simulink model "Mdl_Gear"  (R2024b)
settings: Solver=FixedStepDiscrete  StartTime=0.0  StopTime=10.0  FixedStep=0.1  RelTol=1e-3  EnableMultiTasking=on
values from neighbouring files (symbols this model uses):
  GEAR_MODE_OFF = mpt.Parameter    [Mdl_Gear_DD.m]
  GEAR_STATUS_OFF = mpt.Parameter    [Mdl_Gear_DD.m]
  HMI_READY = mpt.Parameter    [Mdl_Gear_DD.m]
  IND_FLASH_1HZ = mpt.Parameter    [Mdl_Gear_DD.m]
  IND_FLASH_4HZ = mpt.Parameter    [Mdl_Gear_DD.m]
  IND_TURN_OFF = mpt.Parameter    [Mdl_Gear_DD.m]
  Init_Count = mpt.Parameter    [Mdl_Gear_DD.m]
  Mdl_Gear_cTaskPeriod = mpt.Parameter    [Mdl_Gear_rte_types.m]
  PGM_LOGIC_ENABLE = mpt.Parameter    [Mdl_Gear_DD.m]
  RTE_E_MAX_AGE_EXCEEDED = mpt.Parameter    [Mdl_Gear_rte_types.m]
  RTE_E_NEVER_RECEIVED = mpt.Parameter    [Mdl_Gear_rte_types.m]
  Shift_Blink_P1 = mpt.Parameter    [Mdl_Gear_DD.m]
  Shift_Blink_P2 = mpt.Parameter    [Mdl_Gear_DD.m]
  STATUS_OFF = mpt.Parameter    [Mdl_Gear_DD.m]
  STATUS_ON = mpt.Parameter    [Mdl_Gear_DD.m]
  Timer_Param = mpt.Parameter    [Mdl_Gear_DD.m]
  TYPE1 = mpt.Parameter    [Mdl_Gear_DD.m]
  TYPE1_SBW = mpt.Parameter    [Mdl_Gear_DD.m]
  TYPE2 = mpt.Parameter    [Mdl_Gear_DD.m]
  TYPE2_MECH = mpt.Parameter    [Mdl_Gear_DD.m]
  TYPE3 = mpt.Parameter    [Mdl_Gear_DD.m]
  VALUE_FIFTEEN = mpt.Parameter    [Mdl_Gear_DD.m]
  VALUE_FIVE = mpt.Parameter    [Mdl_Gear_DD.m]
  VALUE_FOUR = mpt.Parameter    [Mdl_Gear_DD.m]
  VALUE_ONE = mpt.Parameter    [Mdl_Gear_DD.m]
  VALUE_TEN = mpt.Parameter    [Mdl_Gear_DD.m]
  VALUE_THREE = mpt.Parameter    [Mdl_Gear_DD.m]
  VALUE_TWO = mpt.Parameter    [Mdl_Gear_DD.m]
  VALUE_ZERO = mpt.Parameter    [Mdl_Gear_DD.m]
undefined symbols (not defined in the file or in its folder): CLUSTER_INACTIVE, eGearIn, eGearModeIn, eGearRecommendationIn, eGearStatusIn, eSIGNAL_MISSING, eSIGNAL_NEVER_RECEIVED, IgnOff, IgnOn, NETWORK_NORMAL, NETWORK_STANDALONE, PTSYS_EV, PTSYS_PHV, tRxSignalId_type_instance, tRxSignalStatus_type_instance
libraries: simulink x9
(part 2 of 2)

== matlab function Mdl_Gear/Mdl_Gear_Task_sys/Subsystem/Subsystem1/Subsystem/Display Blink Effect Determination ==
  data: Vehicle_status input; GearStatus_Val input; IND_FLASH_4HZ parameter; IND_FLASH_1HZ parameter; Shift_Blink_Pattern output; IND_TURN_OFF parameter; Shift_Blink_P2 parameter; Shift_Blink_P1 parameter; GEAR_MODE_OFF parameter; GearStatus_Sts input; eSIGNAL_NEVER_RECEIVED parameter; eSIGNAL_MISSING parameter; Prev_Shift_Blink_Pattern input; NETWORK_STANDALONE parameter
function Shift_Blink_Pattern = fcn(Vehicle_status, GearStatus_Val, IND_FLASH_4HZ, IND_FLASH_1HZ, IND_TURN_OFF, Shift_Blink_P2, Shift_Blink_P1, GEAR_MODE_OFF, GearStatus_Sts, eSIGNAL_NEVER_RECEIVED, eSIGNAL_MISSING, Prev_Shift_Blink_Pattern, NETWORK_STANDALONE)

aVarTruthTableCondition_1 = false;
aVarTruthTableCondition_2 = false;
aVarTruthTableCondition_3 = false;
aVarTruthTableCondition_4 = false;


% Appmode is Standalone or  CAN status is never recived

aVarTruthTableCondition_1 = logical(((Vehicle_status == NETWORK_STANDALONE ) || ( GearStatus_Sts == eSIGNAL_NEVER_RECEIVED)));

% Blink_Pattern Off

aVarTruthTableCondition_2 = logical(( GearStatus_Sts== eSIGNAL_MISSING));

% Blink Pattern 1

aVarTruthTableCondition_3 = logical(GearStatus_Val== Shift_Blink_P1);

% Blink Pattern 2

aVarTruthTableCondition_4 = logical(GearStatus_Val== Shift_Blink_P2);

if (aVarTruthTableCondition_1)
    aFcnTruthTableAction_4();
elseif (aVarTruthTableCondition_2)
    aFcnTruthTableAction_1();
elseif (aVarTruthTableCondition_3)
    aFcnTruthTableAction_2();
elseif (aVarTruthTableCondition_4)
    aFcnTruthTableAction_3();
else % Default
    aFcnTruthTableAction_1();
end

function aFcnTruthTableAction_1()

% Shift Blink OFF

Shift_Blink_Pattern = IND_TURN_OFF;

function aFcnTruthTableAction_2()

% Shift Blink Pattern 1 as 1 Hz

Shift_Blink_Pattern = IND_FLASH_1HZ;

function aFcnTruthTableAction_3()

% Shift Blink Pattern 2 as 4 hz

Shift_Blink_Pattern = IND_FLASH_4HZ;

function aFcnTruthTableAction_4()

% No change

Shift_Blink_Pattern = Prev_Shift_Blink_Pattern;

== matlab function Mdl_Gear/Mdl_Gear_Task_sys/Subsystem/Subsystem1/Subsystem/Determination of Shift Up ==
  data: Vehicle_status input; Shift_Up_Ind output; STATUS_OFF parameter; Shift_Up_Can_Value input; Shift_Up_Can_Status input; NETWORK_NORMAL parameter; NETWORK_STANDALONE parameter; eSIGNAL_NEVER_RECEIVED parameter; eSIGNAL_MISSING parameter; Prev_Shift_Up_Ind input; VALUE_ONE parameter; VALUE_FIFTEEN parameter; STATUS_ON parameter
function Shift_Up_Ind = fcn(Vehicle_status, STATUS_OFF, Shift_Up_Can_Value, Shift_Up_Can_Status, NETWORK_NORMAL, NETWORK_STANDALONE, eSIGNAL_NEVER_RECEIVED, eSIGNAL_MISSING, Prev_Shift_Up_Ind, VALUE_ONE, VALUE_FIFTEEN, STATUS_ON)

aVarTruthTableCondition_1 = false;
aVarTruthTableCondition_2 = false;
aVarTruthTableCondition_3 = false;


% Appmode is Standalone or  CAN status is never recived

aVarTruthTableCondition_1 = logical(((Vehicle_status == NETWORK_STANDALONE ) || ( Shift_Up_Can_Status == eSIGNAL_NEVER_RECEIVED)));

% CAN status is Missing

aVarTruthTableCondition_2 = logical((Shift_Up_Can_Status == eSIGNAL_MISSING));

% Shift Up CAN value is 1

aVarTruthTableCondition_3 = logical((Shift_Up_Can_Value == VALUE_ONE));

if (aVarTruthTableCondition_1)
    aFcnTruthTableAction_2();
elseif (aVarTruthTableCondition_2)
    aFcnTruthTableAction_1();
elseif (aVarTruthTableCondition_3)
    aFcnTruthTableAction_3();
else % Default
    aFcnTruthTableAction_1();
end

function aFcnTruthTableAction_1()

% Shift up is Off

Shift_Up_Ind = STATUS_OFF;

function aFcnTruthTableAction_2()

% Previous Step Up

Shift_Up_Ind = Prev_Shift_Up_Ind;

function aFcnTruthTableAction_3()

% Shift up is On

Shift_Up_Ind = STATUS_ON;

== matlab function Mdl_Gear/Mdl_Gear_Task_sys/Subsystem/Subsystem1/Subsystem/Determination of Shift Down ==
  data: Vehicle_status input; Shift_Down_Ind output; STATUS_OFF parameter; Shift_Down_Can_Value input; Shift_Down_Can_Status input; NETWORK_NORMAL parameter; NETWORK_STANDALONE parameter; eSIGNAL_NEVER_RECEIVED parameter; eSIGNAL_MISSING parameter; Prev_Shift_Down_Ind input; VALUE_TWO parameter; VALUE_FIFTEEN parameter; STATUS_ON parameter
function Shift_Down_Ind = fcn(Vehicle_status, STATUS_OFF, Shift_Down_Can_Value, Shift_Down_Can_Status, NETWORK_NORMAL, NETWORK_STANDALONE, eSIGNAL_NEVER_RECEIVED, eSIGNAL_MISSING, Prev_Shift_Down_Ind, VALUE_TWO, VALUE_FIFTEEN, STATUS_ON)

aVarTruthTableCondition_1 = false;
aVarTruthTableCondition_2 = false;
aVarTruthTableCondition_3 = false;


% Appmode is Standalone or  CAN status is never recived

aVarTruthTableCondition_1 = logical(((Vehicle_status == NETWORK_STANDALONE ) || ( Shift_Down_Can_Status == eSIGNAL_NEVER_RECEIVED)));

% CAN status is Missing

aVarTruthTableCondition_2 = logical((Shift_Down_Can_Status == eSIGNAL_MISSING));

% Shift down CAN value is 1

aVarTruthTableCondition_3 = logical((Shift_Down_Can_Value == VALUE_TWO));

if (aVarTruthTableCondition_1)
    aFcnTruthTableAction_2();
elseif (aVarTruthTableCondition_2)
    aFcnTruthTableAction_1();
elseif (aVarTruthTableCondition_3)
    aFcnTruthTableAction_3();
else % Default
    aFcnTruthTableAction_1();
end

function aFcnTruthTableAction_1()

% Shift down status is Off

Shift_Down_Ind = STATUS_OFF;

function aFcnTruthTableAction_2()

% Previous Shift down status

Shift_Down_Ind = Prev_Shift_Down_Ind;

function aFcnTruthTableAction_3()

% Shift down status is On

Shift_Down_Ind = STATUS_ON;

== matlab function Mdl_Gear/Mdl_Gear_Task_sys/Subsystem/Subsystem1/Subsystem/Determination of Display deceleration state ==
  data: Vehicle_status input; PTSys_flag input; DisplayDecState output; STATUS_OFF parameter; SFT_MET_Value input; SFT_MET_Status input; CLDCLV_Value input; CLDCLV_Status input; NETWORK_NORMAL parameter; NETWORK_STANDALONE parameter; RTE_E_NEVER_RECEIVED parameter; RTE_E_MAX_AGE_EXCEEDED parameter; Prev_DisplayDecState input; VALUE_ONE parameter; VALUE_TWO parameter; VALUE_ZERO parameter; VALUE_THREE parameter; VALUE_FOUR parameter; VALUE_FIVE parameter; PTSYS_PHV parameter; PTSYS_EV parameter
function DisplayDecState = fcn(Vehicle_status, PTSys_flag, STATUS_OFF, SFT_MET_Value, SFT_MET_Status, CLDCLV_Value, CLDCLV_Status, NETWORK_NORMAL, NETWORK_STANDALONE, RTE_E_NEVER_RECEIVED, RTE_E_MAX_AGE_EXCEEDED, Prev_DisplayDecState, VALUE_ONE, VALUE_TWO, VALUE_ZERO, VALUE_THREE, VALUE_FOUR, VALUE_FIVE, PTSYS_PHV, PTSYS_EV)

aVarTruthTableCondition_1 = false;
aVarTruthTableCondition_2 = false;
aVarTruthTableCondition_3 = false;
aVarTruthTableCondition_4 = false;
aVarTruthTableCondition_5 = false;
aVarTruthTableCondition_6 = false;
aVarTruthTableCondition_7 = false;
aVarTruthTableCondition_8 = false;


% Check App mode is Standalone

aVarTruthTableCondition_1 = logical((Vehicle_status == NETWORK_STANDALONE ));

% Check PTsys flag and SFT_MET value is other than 4 and 5

aVarTruthTableCondition_2 = logical((((PTSys_flag ~= PTSYS_PHV) && (PTSys_flag ~= PTSYS_EV)) || ((SFT_MET_Value ~= VALUE_FOUR) && ( SFT_MET_Value ~= VALUE_FIVE))));

% Missing and Never received

aVarTruthTableCondition_3 = logical((CLDCLV_Status == RTE_E_NEVER_RECEIVED) || (CLDCLV_Status == RTE_E_MAX_AGE_EXCEEDED) || (SFT_MET_Status == RTE_E_NEVER_RECEIVED) || (SFT_MET_Status == RTE_E_MAX_AGE_EXCEEDED));

% CANSignal  CLDCLV is 1

aVarTruthTableCondition_4 = logical((CLDCLV_Value == VALUE_ONE));

% CANSignal  CLDCLV is 2

aVarTruthTableCondition_5 = logical((CLDCLV_Value == VALUE_TWO));

% CANSignal  CLDCLV is 3

aVarTruthTableCondition_6 = logical((CLDCLV_Value == VALUE_THREE));

% CANSignal  CLDCLV is 4

aVarTruthTableCondition_7 = logical((CLDCLV_Value == VALUE_FOUR));

% CANSignal  CLDCLV is 5

aVarTruthTableCondition_8 = logical((CLDCLV_Value == VALUE_FIVE));

if (aVarTruthTableCondition_1)
    aFcnTruthTableAction_2();
elseif (aVarTruthTableCondition_2)
    aFcnTruthTableAction_1();
elseif (aVarTruthTableCondition_3)
    aFcnTruthTableAction_1();
elseif (aVarTruthTableCondition_4)
    aFcnTruthTableAction_3();
elseif (aVarTruthTableCondition_5)
    aFcnTruthTableAction_4();
elseif (aVarTruthTableCondition_6)
    aFcnTruthTableAction_5();
elseif (aVarTruthTableCondition_7)
    aFcnTruthTableAction_6();
elseif (aVarTruthTableCondition_8)
    aFcnTruthTableAction_7();
else % Default
    aFcnTruthTableAction_1();
end

function aFcnTruthTableAction_1()

% Off state

DisplayDecState = STATUS_OFF;

function aFcnTruthTableAction_2()

% Previous state

DisplayDecState = Prev_DisplayDecState;

function aFcnTruthTableAction_3()

% LEVEL_0

DisplayDecState = VALUE_ONE;

function aFcnTruthTableAction_4()

% LEVEL_1

DisplayDecState = VALUE_TWO;

function aFcnTruthTableAction_5()

% LEVEL_2

DisplayDecState = VALUE_THREE;

function aFcnTruthTableAction_6()

% LEVEL_3

DisplayDecState = VALUE_FOUR;

function aFcnTruthTableAction_7()

% LEVEL_4

DisplayDecState = VALUE_FIVE;

== matlab function Mdl_Gear/Mdl_Gear_Task_sys/Subsystem/Subsystem1/Subsystem/Output of GUI_SHIFT_TYPE ==
  data: DisplayDecState input; Screen_ShiftType output; STATUS_OFF parameter; Shift_Up_Ind input; Shift_Down_Ind input; VALUE_ONE parameter; VALUE_FIFTEEN parameter; VALUE_FIVE parameter; TYPE1 parameter; TYPE2 parameter; TYPE3 parameter; STATUS_ON parameter
function Screen_ShiftType = fcn(DisplayDecState, STATUS_OFF, Shift_Up_Ind, Shift_Down_Ind, VALUE_ONE, VALUE_FIFTEEN, VALUE_FIVE, TYPE1, TYPE2, TYPE3, STATUS_ON)

aVarTruthTableCondition_1 = false;
aVarTruthTableCondition_2 = false;


% Display Deceleration status is Off and Shift up or Down is On

aVarTruthTableCondition_1 = logical(((DisplayDecState == STATUS_OFF)  && ((Shift_Up_Ind == STATUS_ON) || (Shift_Down_Ind == STATUS_ON))));

% Display Deceleration status is 1 to 5

aVarTruthTableCondition_2 = logical(((DisplayDecState >= VALUE_ONE) && (DisplayDecState <= VALUE_FIVE)));

if (aVarTruthTableCondition_1)
    aFcnTruthTableAction_2();
elseif (aVarTruthTableCondition_2)
    aFcnTruthTableAction_3();
else % Default
    aFcnTruthTableAction_1();
end

function aFcnTruthTableAction_1()

% Screen Shift type is TYPE1

Screen_ShiftType = TYPE1;

function aFcnTruthTableAction_2()

% Screen Shift type is TYPE2

Screen_ShiftType = TYPE2;

function aFcnTruthTableAction_3()

% Screen Shift type is TYPE3

Screen_ShiftType = TYPE3;

== matlab function Mdl_Gear/Mdl_Gear_Task_sys/Subsystem/Subsystem1/Subsystem/Determination of Shift Position and Shift Mode and Gear Step ==
  data: GEAR_STATUS_OFF parameter; Shift_Position input; Shift_Ind_Pos output uint8; Gear_Step input; Shift_Pos_RANGE_P parameter; Shift_Pos_RANGE_R parameter; Shift_Pos_RANGE_N parameter; Shift_Pos_RANGE_B parameter; Shift_Pos_RANGE_SD parameter; Shift_Pos_RANGE_D parameter; Shift_Pos_RANGE_S parameter; Shift_Pos_RANGE_M parameter; Shift_PosInd_Ind_S parameter; Shift_PosInd_Ind_M parameter; Shift_PosInd_Ind_D parameter; Shift_PosInd_P parameter; Shift_PosInd_R parameter; Shift_PosInd_N parameter; Shift_PosInd_D parameter; Shift_PosInd_B parameter; Shift_PosInd_SD parameter; Shift_PosInd_M parameter; Shift_PosInd_S parameter; GEAR_STATUS_ON parameter; Gear_Flag output uint8
function [Shift_Ind_Pos, Gear_Flag] = fcn(GEAR_STATUS_OFF, Shift_Position, Gear_Step, Shift_Pos_RANGE_P, Shift_Pos_RANGE_R, Shift_Pos_RANGE_N, Shift_Pos_RANGE_B, Shift_Pos_RANGE_SD, Shift_Pos_RANGE_D, Shift_Pos_RANGE_S, Shift_Pos_RANGE_M, Shift_PosInd_Ind_S, Shift_PosInd_Ind_M, Shift_PosInd_Ind_D, Shift_PosInd_P, Shift_PosInd_R, Shift_PosInd_N, Shift_PosInd_D, Shift_PosInd_B, Shift_PosInd_SD, Shift_PosInd_M, Shift_PosInd_S, GEAR_STATUS_ON)

aVarTruthTableCondition_1 = false;
aVarTruthTableCondition_2 = false;
aVarTruthTableCondition_3 = false;
aVarTruthTableCondition_4 = false;
aVarTruthTableCondition_5 = false;
aVarTruthTableCondition_6 = false;
aVarTruthTableCondition_7 = false;
aVarTruthTableCondition_8 = false;
aVarTruthTableCondition_9 = false;
aVarTruthTableCondition_10 = false;
aVarTruthTableCondition_11 = false;
aVarTruthTableCondition_12 = false;
aVarTruthTableCondition_13 = false;


% Shift Position Determination Range P,R,N,B,SD and Gear Step >0

aVarTruthTableCondition_1 = logical(((Shift_Position == Shift_Pos_RANGE_P)||(Shift_Position == Shift_Pos_RANGE_N)||(Shift_Position == Shift_Pos_RANGE_R)|| (Shift_Position == Shift_Pos_RANGE_B)||(Shift_Position == Shift_Pos_RANGE_SD)) &&(Gear_Step == GEAR_STATUS_OFF));

% Shift Position Determination Range P and Gear Step ==0

aVarTruthTableCondition_2 = logical((Shift_Position== Shift_Pos_RANGE_P));

% Shift Position Determination Range R and Gear Step ==0

aVarTruthTableCondition_3 = logical((Shift_Position == Shift_Pos_RANGE_R));

% Shift Position Determination Range N and Gear Step ==0

aVarTruthTableCondition_4 = logical((Shift_Position == Shift_Pos_RANGE_N));

% Shift Position Determination Range D and Gear Step ==0

aVarTruthTableCondition_5 = logical((Shift_Position == Shift_Pos_RANGE_D));

% Shift Position Determination Range B and Gear Step ==0

aVarTruthTableCondition_6 = logical((Shift_Position == Shift_Pos_RANGE_B));

% Shift Position Determination Range SD and Gear Step ==0

aVarTruthTableCondition_7 = logical((Shift_Position == Shift_Pos_RANGE_SD));

% Shift Position Determination M and Gear Step 0

aVarTruthTableCondition_8 = logical((Shift_Position == Shift_Pos_RANGE_M)&&(Gear_Step ==GEAR_STATUS_OFF));

% Shift Position Determination M and Gear Step >0

aVarTruthTableCondition_9 = logical((Shift_Position == Shift_Pos_RANGE_M)&&(Gear_Step >GEAR_STATUS_OFF));

% Shift Position Determination S and Gear Step =0

aVarTruthTableCondition_10 = logical((Shift_Position == Shift_Pos_RANGE_S)&&(Gear_Step ==GEAR_STATUS_OFF));

% Shift Position Determination S and Gear Step >0

aVarTruthTableCondition_11 = logical((Shift_Position == Shift_Pos_RANGE_S)&&(Gear_Step >GEAR_STATUS_OFF));

% Shift Position Determination D and Gear Step 0

aVarTruthTableCondition_12 = logical((Shift_Position == Shift_Pos_RANGE_D)&&(Gear_Step ==GEAR_STATUS_OFF));

% Shift Position Determination D and Gear Step >0

aVarTruthTableCondition_13 = logical((Shift_Position == Shift_Pos_RANGE_D)&&(Gear_Step > GEAR_STATUS_OFF));

if (aVarTruthTableCondition_1)
    aFcnTruthTableAction_1();
elseif (aVarTruthTableCondition_2)
    aFcnTruthTableAction_2();
elseif (aVarTruthTableCondition_3)
    aFcnTruthTableAction_3();
elseif (aVarTruthTableCondition_4)
    aFcnTruthTableAction_4();
elseif (aVarTruthTableCondition_6)
    aFcnTruthTableAction_5();
elseif (aVarTruthTableCondition_7)
    aFcnTruthTableAction_6();
elseif (aVarTruthTableCondition_8)
    aFcnTruthTableAction_9();
elseif (aVarTruthTableCondition_9)
    aFcnTruthTableAction_10();
elseif (aVarTruthTableCondition_10)
    aFcnTruthTableAction_11();
elseif (aVarTruthTableCondition_11)
    aFcnTruthTableAction_12();
elseif (aVarTruthTableCondition_5 && aVarTruthTableCondition_12)
    aFcnTruthTableAction_7();
elseif (aVarTruthTableCondition_13)
    aFcnTruthTableAction_8();
else % Default
    aFcnTruthTableAction_1();
end

function aFcnTruthTableAction_1()

% Shift Position Determination OFF

Shift_Ind_Pos = GEAR_STATUS_OFF;
Gear_Flag = GEAR_STATUS_OFF;

function aFcnTruthTableAction_2()

% Shift Position Determination Range P and Gear Step  0

Shift_Ind_Pos = Shift_PosInd_P;
Gear_Flag = GEAR_STATUS_OFF;

function aFcnTruthTableAction_3()

% Shift Position Determination Range R and Gear Step  0

Shift_Ind_Pos = Shift_PosInd_R;
Gear_Flag = GEAR_STATUS_OFF;

function aFcnTruthTableAction_4()

% Shift Position Determination Range N and Gear Step  0

Shift_Ind_Pos = Shift_PosInd_N;
Gear_Flag = GEAR_STATUS_OFF;

function aFcnTruthTableAction_5()

% Shift Position Determination Range B and Gear Step  0

Shift_Ind_Pos = Shift_PosInd_B;
Gear_Flag = GEAR_STATUS_OFF;

function aFcnTruthTableAction_6()

% Shift Position Determination Range SD and Gear Step  0

Shift_Ind_Pos = Shift_PosInd_SD;
Gear_Flag = GEAR_STATUS_OFF;

function aFcnTruthTableAction_7()

% Shift Position Determination Range D and Gear Step  0

Shift_Ind_Pos = Shift_PosInd_D;
Gear_Flag = GEAR_STATUS_OFF;

function aFcnTruthTableAction_8()

% Shift Position Determination Range D and Gear Step  > 0

Shift_Ind_Pos = Shift_PosInd_D;
Gear_Flag = GEAR_STATUS_ON;

function aFcnTruthTableAction_9()

% Shift Position Determination Range M and Gear Step 0

Shift_Ind_Pos = Shift_PosInd_M;
Gear_Flag = GEAR_STATUS_OFF;

function aFcnTruthTableAction_10()

% Shift Position Determination Range M and Gear Step >0

Shift_Ind_Pos = Shift_PosInd_M;
Gear_Flag = GEAR_STATUS_ON;

function aFcnTruthTableAction_11()

% Shift Position Determination Range S and Gear Step 0

Shift_Ind_Pos = Shift_PosInd_S;
Gear_Flag = GEAR_STATUS_OFF;

function aFcnTruthTableAction_12()

% Shift Position Determination Range S and Gear Step >0

Shift_Ind_Pos = Shift_PosInd_S;
Gear_Flag = GEAR_STATUS_ON;

== matlab function Mdl_Gear/Mdl_Gear_Task_sys/Subsystem/Subsystem1/Subsystem/CAN Signal Determination for Shift Type/Shift Position Up Down CAN Signal Determination ==
  data: GEAR_Type_SEL input uint8; Gear_Val input uint8; Gear_Sts input uint8; GearRcmd_Val input uint8; GearRcmd_Sts input uint8; GearStatus_Val input uint8; GearStatus_Sts input uint8; TYPE1_SBW parameter; Shift_Position_Can_Value output uint8; Shift_Position_Can_Status output uint8; Shift_Up_Can_Value output uint8; Shift_Up_Can_Status output uint8; Shift_Down_Can_Value output uint8; Shift_Down_Can_Status output uint8
function [Shift_Position_Can_Value, Shift_Position_Can_Status, Shift_Up_Can_Value, Shift_Up_Can_Status, Shift_Down_Can_Value, Shift_Down_Can_Status] = tt_blk_kernel(GEAR_Type_SEL, Gear_Val, Gear_Sts, GearRcmd_Val, GearRcmd_Sts, GearStatus_Val, GearStatus_Sts, TYPE1_SBW)

aVarTruthTableCondition_1 = false;


% Check Shift type 1 or 2

aVarTruthTableCondition_1 = logical(GEAR_Type_SEL == TYPE1_SBW);

if (aVarTruthTableCondition_1)
    aFcnTruthTableAction_1();
else % Default
    aFcnTruthTableAction_2();
end

function aFcnTruthTableAction_1()

% Type 1 : SBW

Shift_Position_Can_Value = Gear_Val;
Shift_Position_Can_Status = Gear_Sts;
Shift_Up_Can_Value = GearRcmd_Val;
Shift_Up_Can_Status = GearRcmd_Sts;
Shift_Down_Can_Value = GearRcmd_Val;
Shift_Down_Can_Status = GearRcmd_Sts;

function aFcnTruthTableAction_2()

% Type 2 : Mechanical shift

Shift_Position_Can_Value = Gear_Val;
Shift_Position_Can_Status = Gear_Sts;
Shift_Up_Can_Value = GearRcmd_Val;
Shift_Up_Can_Status = GearRcmd_Sts;
Shift_Down_Can_Value = GearRcmd_Val;
Shift_Down_Can_Status = GearRcmd_Sts;
